simulink model "script_1"  (R2024b)
settings: Solver=VariableStepAuto  StartTime=0.0  StopTime=20  RelTol=1e-3
model workspace (MAT data in the model file):
  A = Simulink.Parameter
  A.Complexity = 'real'
  A.Dimensions = [0 0]
  A.DataType = 'auto'
settings Model: Creator=21609  LastModifiedBy=21609

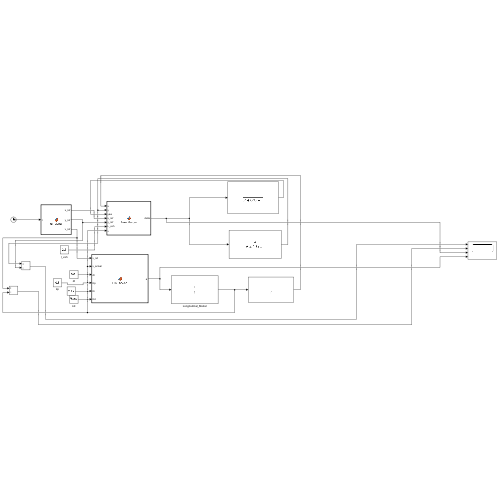
[thumbnail: Simulink's stored preview of the top-level diagram]
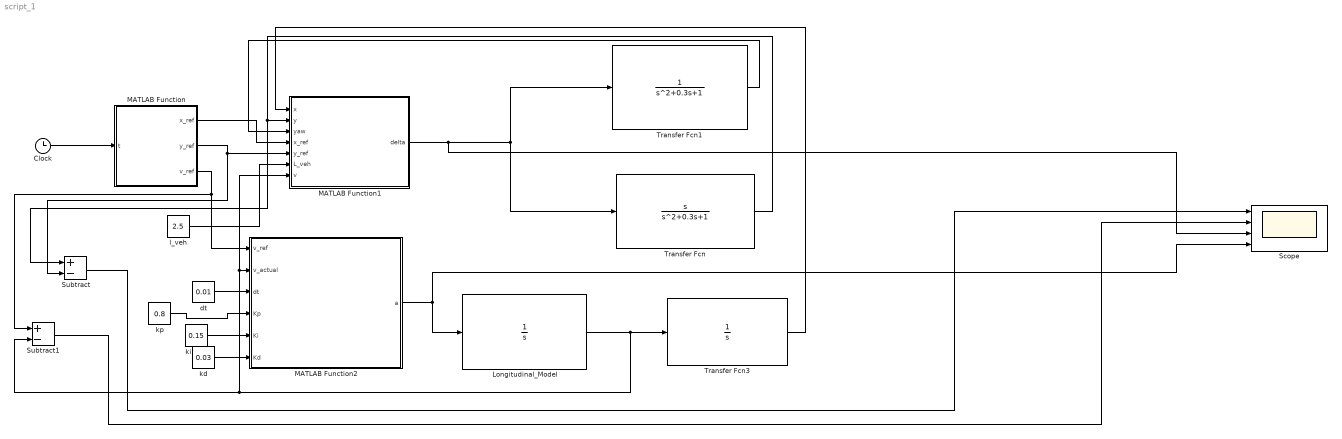
== system script_1 ==
  Clock : Clock
  Longitudinal_Model : TransferFcn  Denominator=[1 0]
  MATLAB Function : MATLAB Function  TreatAsAtomicUnit=on
  MATLAB Function1 : MATLAB Function  TreatAsAtomicUnit=on
  MATLAB Function2 : MATLAB Function  TreatAsAtomicUnit=on
  Scope : Scope  NumInputPorts=4
  Subtract : Sum  Inputs=+-
  Subtract1 : Sum  Inputs=+-
  Transfer Fcn : TransferFcn  Numerator=[1 0]  Denominator=[1 0.3 1]
  Transfer Fcn1 : TransferFcn  Numerator=[0 1]  Denominator=[1 0.3 1]
  Transfer Fcn3 : TransferFcn  Denominator=[1 0]
  dt : Constant  Value=0.01
  kd : Constant  Value=0.03
  ki : Constant  Value=0.15
  kp : Constant  Value=0.8
  l_veh : Constant  Value=2.5
  wires:
  Clock/1 -> MATLAB Function/1(t)
  Longitudinal_Model/1 -> Transfer Fcn3/1, Subtract1/2, MATLAB Function1/7(v), MATLAB Function2/2(v_actual)
  dt/1 -> MATLAB Function2/3(dt)
  kd/1 -> MATLAB Function2/6(Kd)
  ki/1 -> MATLAB Function2/5(Ki)
  kp/1 -> MATLAB Function2/4(Kp)
  l_veh/1 -> MATLAB Function1/6(L_veh)
  MATLAB Function/1(x_ref) -> MATLAB Function1/4(x_ref)
  MATLAB Function/2(y_ref) -> Subtract/2, MATLAB Function1/5(y_ref)
  MATLAB Function/3(v_ref) -> MATLAB Function2/1(v_ref), Subtract1/1
  Transfer Fcn3/1 -> MATLAB Function1/1(x)
  Transfer Fcn/1 -> Subtract/1, MATLAB Function1/2(y)
  Transfer Fcn1/1 -> MATLAB Function1/3(yaw)
  MATLAB Function1/1(delta) -> Scope/3, Transfer Fcn/1, Transfer Fcn1/1
  MATLAB Function2/1(a) -> Longitudinal_Model/1, Scope/4
  Subtract/1 -> Scope/1
  Subtract1/1 -> Scope/2

== matlab function script_1/MATLAB Function1 ==
  data: x input; delta output; y input; yaw input; x_ref input; y_ref input; L_veh input; v input
function delta = Pure_Pursuit(x, y, yaw, x_ref, y_ref, L_veh, v)
    % 输入：车辆状态（x,y,yaw,v）、参考点（x_ref,y_ref）、轴距L_veh
    % 输出：转向角delta（标量，限幅±0.52rad≈30°）
    L = 1.5 + 0.4*v;  % 预瞄距离（与速度正相关）
    L = max(L, 2);    % 最小预瞄距离2m
    
    % 计算车辆到参考点的横向距离（标量运算）
    dx = x_ref - x;
    dy = y_ref - y;
    dy_veh = -dx*sin(yaw) + dy*cos(yaw);  % 车辆坐标系下横向距离
    
    % 计算转向角并限幅
    delta = atan2(2*L_veh*dy_veh, L^2);
    delta = max(min(delta, 0.52), -0.52);
end

== matlab function script_1/MATLAB Function ==
  data: t input; x_ref output; y_ref output; v_ref output
function [x_ref, y_ref, v_ref] = ref_signal(t)
    % 输入：t（仿真时间，标量）
    % 输出：当前参考点（x_ref,y_ref）和参考速度v_ref（均为标量）
    if t <= 10  % 0-10s：直线（y=0）
        x_ref = 8*t;    % 纵向位置随时间增加（8m/s）
        y_ref = 0;      % 横向位置为0
        v_ref = 8;      % 参考速度8m/s
    else        % 10s后：圆弧（半径40m）
        theta = (t-10)/4;  % 角度随时间变化
        x_ref = 80 + 40*sin(theta);  % 圆弧x坐标
        y_ref = 40 - 40*cos(theta);  % 圆弧y坐标
        v_ref = 6;      % 弯道减速到6m/s
    end
end

== matlab function script_1/MATLAB Function2 ==
  settings: updateMethod=DISCRETE
  data: v_ref input; a output; v_actual input; dt input; Kp input; Ki input; Kd input
function a = PID_Speed(v_ref, v_actual, dt, Kp, Ki, Kd)
    % 输入：参考速度v_ref、实际速度v_actual、步长dt、PID参数
    % 输出：加速度a（标量，限幅±2m/s²）
    persistent integral e_prev  % 积分项和上一时刻偏差
    if isempty(integral), integral = 0; e_prev = 0; end
    
    e = v_ref - v_actual;  % 速度偏差
    integral = integral + e*dt;  % 积分项（无死区，简化）
    integral = max(min(integral, 5), -5);  % 积分限幅
    derivative = (e - e_prev)/dt;  % 微分项
    e_prev = e;
    
    a = Kp*e + Ki*integral + Kd*derivative;  % PID输出
    a = max(min(a, 2), -2);  % 加速度限幅
end
